simulink model "eom"  (R2021b)
settings: Solver=ode4  StartTime=0.0  StopTime=100  RelTol=1e-3  EnableMultiTasking=on
PreLoadFcn:
  | PARAMETROS
values from neighbouring files (symbols this model uses):
  b = 0.353    [PARAMETROS.m]    (also in forandtor.m; forandtorPARAM.m)
  CDfront = 0.5    [PARAMETROS.m]    (also in forandtor.m; forandtorPARAM.m)
  CDlat = 0.75    [PARAMETROS.m]    (also in forandtor.m; forandtorPARAM.m)
  CLa = 1    [PARAMETROS.m]    (also in forandtor.m; forandtorPARAM.m)
  CLp = 5    [PARAMETROS.m]    (also in forandtor.m; forandtorPARAM.m)
  CMdeltae = 1    [PARAMETROS.m]    (also in forandtor.m; forandtorPARAM.m)
  CMfq = 1    [PARAMETROS.m]    (also in forandtor.m; forandtorPARAM.m)
  CMw = 10    [PARAMETROS.m]    (also in forandtor.m; forandtorPARAM.m)
  CNdeltar = 1    [PARAMETROS.m]    (also in forandtor.m; forandtorPARAM.m)
  CNfr = 1    [PARAMETROS.m]    (also in forandtor.m; forandtorPARAM.m)
  CNv = 10    [PARAMETROS.m]    (also in forandtor.m; forandtorPARAM.m)
  fullt = 600    [PARAMETROS.m]    (also in forandtor.m; forandtorPARAM.m)
  g = 9.81    [PARAMETROS.m]    (also in eom1.m; eom1PARAM.m)
  Ix = 0.468    [PARAMETROS.m]    (also in eom1.m; eom1PARAM.m)
  Iy = 90.8    [PARAMETROS.m]    (also in eom1.m; eom1PARAM.m)
  Iz = Iy    (= 90.8)    [PARAMETROS.m]    (also in eom1.m; eom1PARAM.m)
  m = 85.3    [PARAMETROS.m]    (also in eom1.m; eom1PARAM.m)
  Sfront = 0.0127    [PARAMETROS.m]    (also in forandtor.m; forandtorPARAM.m)
  Slat = 1.2049    [PARAMETROS.m]    (also in forandtor.m; forandtorPARAM.m)
  Sstab = 0.45    [PARAMETROS.m]    (also in forandtor.m; forandtorPARAM.m)
  Swing = 0.4525    [PARAMETROS.m]    (also in forandtor.m; forandtorPARAM.m)
libraries: aerolibanim x6, aerolibatmos2 x3
(part 1 of 2)
settings Model: Creator=verti  LastModifiedBy=patri
settings SolverCC: MaxConsecutiveMinStep=0.1  ZeroCrossAlgorithm=Adaptive  AlgebraicLoopSolver=TrustRegion  AutoInsertRateTranBlk=on
settings DataIOCC: LimitDataPoints=on  ReturnWorkspaceOutputs=off
settings OptimizationCC: LifeSpan=inf
settings DebuggingCC: MultiTaskRateTransMsg=warning  AllowSymbolicDim=off  SFUnexpectedBacktrackingDiag=warning  SFNoUnconditionalDefaultTransitionDiag=warning  SFExecutionAtInitializationDiag=none  SFMachineParentedDataDiag=warning  ArithmeticOperatorsInVariantConditions=warning
settings ModelReferenceCC: PropagateSignalLabelsOutOfModel=off
settings SFSimCC: SimUseLocalCustomCode=off  CustomCodeUndefinedFunction=UseInterfaceOnly
settings RTWCC: RTWUseLocalCustomCode=off
settings CodeAppCC: StateflowObjectComments=on
settings GRTTargetCC: TargetLangStandard=C89/C90 (ANSI)
settings ConfigComp: CovMetricSettings=dw  CovSaveCumulativeToWorkspaceVar=on  CovSaveSingleToWorkspaceVar=on  CovExternalEMLEnable=off

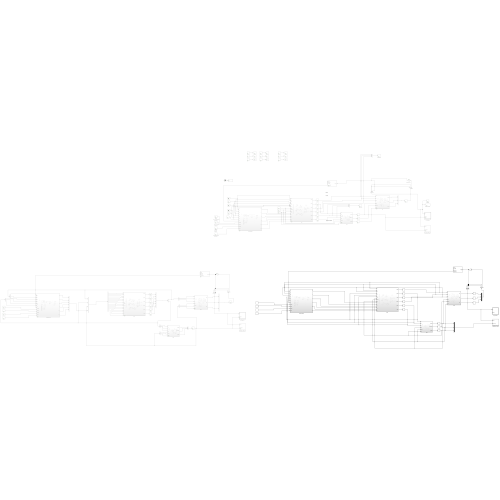
[thumbnail: Simulink's stored preview of the top-level diagram]
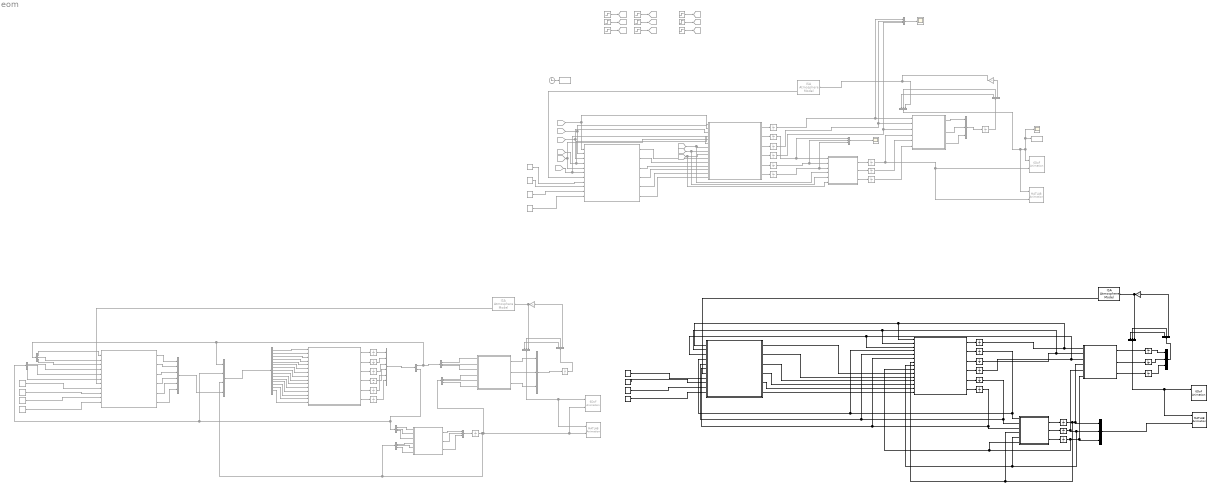
== system eom ==
  note: x,y,z
  note: Ángulos de Euler
  note: P,Q,R
  note: U,V,W
  Animación para ver la posición : aerolibanim/6DoF Animation  Commented=on  u1=[-1000 1000 -1000 1000 0 1300]  u2=0.1  u3=150.0  u4=[4000 0 -5000]  u5=Fixed position  u6=[2000 500 -3150]  u7=10  u8=on
  Animación para ver la posición1 : aerolibanim/6DoF Animation  Commented=on  u1=[-1000 1000 -1000 1000 0 1300]  u2=0.1  u3=150.0  u4=[4000 0 -5000]  u5=Fixed position  u6=[2000 500 -3150]  u7=10  u8=on
  Animación para ver la posición2 : aerolibanim/6DoF Animation  u1=[-1000 1000 -1000 1000 0 1300]  u2=0.1  u3=150.0  u4=[4000 0 -5000]  u5=Fixed position  u6=[2000 500 -3150]  u7=10  u8=on
  Animación para ver ángulos de euler : aerolibanim/MATLAB Animation  Tag=Matlab Animation 6 DOF  Commented=on  Vehicles=1  Geometries='astredwedge.mat'  BoundingBoxCoordinates=[-50,50,-50,50,-50,50]  CameraOffset=[-150,-50,0]  CameraViewAngle=3  SampleTime=0.2  FigurePosition=[1.386000e+02,5.322000e+02,368,2.696000e+02]
      settings: SourceProductBaseCode=AE
  Animación para ver ángulos de euler1 : aerolibanim/MATLAB Animation  Tag=Matlab Animation 6 DOF  Commented=on  Vehicles=1  Geometries='astredwedge.mat'  BoundingBoxCoordinates=[-50,50,-50,50,-50,50]  CameraOffset=[-150,-50,0]  CameraViewAngle=3  SampleTime=0.2  FigurePosition=[1.386000e+02,5.322000e+02,368,2.696000e+02]
      settings: SourceProductBaseCode=AE
  Animación para ver ángulos de euler2 : aerolibanim/MATLAB Animation  Tag=Matlab Animation 6 DOF  Vehicles=1  Geometries='astredwedge.mat'  BoundingBoxCoordinates=[-50,50,-50,50,-50,50]  CameraOffset=[-150,-50,0]  CameraViewAngle=3  SampleTime=0.2  FigurePosition=[1.386000e+02,5.322000e+02,368,2.696000e+02]
      settings: SourceProductBaseCode=AE
  Clock : Clock  Commented=on
  Constant1 : Constant  Value=0.1
  Constant2 : Constant  Commented=on  Value=0.1
  Constant3 : Constant  Commented=on  Value=0
  Constant4 : Constant  Commented=on  Value=0
  Constant5 : Constant  Commented=on
  Constant6 : Constant  Value=0
  Constant7 : Constant  Value=0
  Constant8 : Constant
  Demux{,1..2,5..9} (8 alike) : Demux  Commented=on  Outputs=3
  Demux18 : Demux  Outputs=3
  Demux3 : Demux  Commented=on  Outputs=15
  Demux4 : Demux  Commented=on  Outputs=2
  From1 : From  Commented=on  GotoTag=phi
  From2 : From  Commented=on  GotoTag=psi
  From3 : From  Commented=on  GotoTag=P
  From4 : From  Commented=on  GotoTag=Q
  From5 : From  Commented=on  GotoTag=R
  From6 : From  Commented=on  GotoTag=U
  From7 : From  Commented=on  GotoTag=W
  From8 : From  Commented=on  GotoTag=V
  From9 : From  Commented=on  GotoTag=theta
  Gain : Gain  Commented=on  Gain=-1
  Gain1 : Gain  Gain=-1
  Goto : Goto  Commented=on  GotoTag=U
  Goto1 : Goto  Commented=on  GotoTag=V
  Goto2 : Goto  Commented=on  GotoTag=W
  Goto3 : Goto  Commented=on  GotoTag=P
  Goto4 : Goto  Commented=on  GotoTag=Q
  Goto5 : Goto  Commented=on  GotoTag=R
  Goto6 : Goto  Commented=on  GotoTag=phi
  Goto7 : Goto  Commented=on  GotoTag=theta
  Goto8 : Goto  Commented=on  GotoTag=psi
  ISA Atmosphere Model : aerolibatmos2/ISA Atmosphere Model  Commented=on  custom=off  g=9.80665  gamma=1.4  R=287.0531  L=0.0065  h_trop=11000  h_strat=20000  rho0=1.225  P0=101325  T0=288.15  h0=0
  ISA Atmosphere Model1 : aerolibatmos2/ISA Atmosphere Model  custom=off  g=9.80665  gamma=1.4  R=287.0531  L=0.0065  h_trop=11000  h_strat=20000  rho0=1.225  P0=101325  T0=288.15  h0=0
  ISA Atmosphere Model2 : aerolibatmos2/ISA Atmosphere Model  Commented=on  custom=off  g=9.80665  gamma=1.4  R=287.0531  L=0.0065  h_trop=11000  h_strat=20000  rho0=1.225  P0=101325  T0=288.15  h0=0
  Integrator{,3..7,11,13..17} (12 alike) : Integrator  Commented=on  InitialCondition=[200,0,0,0,0,0]
  Integrator{1,8..9,12} (4 alike) : Integrator  Commented=on  InitialCondition=[0,0,0]
  Integrator10 : Integrator  Commented=on  InitialCondition=[0,0,-3000]
  Integrator18 : Integrator  InitialCondition=[0,0,-3000]
  Integrator{19,21..25} (6 alike) : Integrator  InitialCondition=[200,0,0,0,0,0]
  Integrator2 : Integrator  Commented=on  InitialCondition=[0,0,-3000]
  Integrator20 : Integrator  InitialCondition=[0,0,0]
  Integrator26 : Integrator  InitialCondition=[0,0,0]
  Integrator27 : Integrator  InitialCondition=[0,0,0]
  Integrator28 : Integrator  InitialCondition=[0,0,-3000]
  Integrator29 : Integrator  InitialCondition=[0,0,-3000]
  Inversión eje z : Gain  Commented=on  Gain=-1
  Momentos : Scope  Commented=on
  Mux{,2..3,5,7..9} (7 alike) : Mux  Commented=on  Inputs=3
  Mux1 : Mux  Commented=on  Inputs=6
  Mux10 : Mux  Inputs=3
  Mux11 : Mux  Inputs=3
  Mux14 : Mux  Inputs=3
  Mux4 : Mux  Commented=on
  Mux6 : Mux  Commented=on  Inputs=6
  Palanca de gases Empuje1 : Constant  Commented=on
  Step{,1..8} (9 alike) : Step  Commented=on  SampleTime=0
  To Workspace : ToWorkspace  Commented=on  VariableName=t  SampleTime=-1
  Vector posición : ToWorkspace  Commented=on  VariableName=posicion  SampleTime=-1
      settings: Decimation=2
  Velocidad : Scope  Commented=on
  delta timon profundidad cabeceo1 : Constant  Commented=on  Value=0.1
  deltaa alerones balance1 : Constant  Commented=on  Value=0
  deltar Timon vertical guiñada1 : Constant  Commented=on  Value=0
  eom : Subsystem  Commented=on
  eom1 : Subsystem  Commented=on  ClipboardFcn=PARAMETROS
  eom2 : Subsystem  ClipboardFcn=PARAMETROS
  forcesandtorq : Subsystem  Commented=on
  forcesandtorq1 : Subsystem  Commented=on  ClipboardFcn=PARAMETROS
  forcesandtorq2 : Subsystem  ClipboardFcn=PARAMETROS
  posición : Scope  Commented=on
  rang : Subsystem  Commented=on
  rang1 : Subsystem  Commented=on
  rang2 : Subsystem
  rtra : Subsystem  Commented=on
  rtra1 : Subsystem  Commented=on
  rtra2 : Subsystem
  wires:
  Clock/1 -> To Workspace/1
  Integrator1/1 -> rtra/4(phi), Animación para ver ángulos de euler/2, Animación para ver la posición/2
  Integrator2/1 -> Demux1/1
  Demux1/3 -> Inversión eje z/1
  Inversión eje z/1 -> Mux2/3, ISA Atmosphere Model/1
  ISA Atmosphere Model/4 -> forcesandtorq/7(ro)
  Demux1/1 -> Mux2/1
  Demux1/2 -> Mux2/2
  Mux2/1 -> posición/1, Vector posición/1, Animación para ver la posición/1, Animación para ver ángulos de euler/1
  delta timon profundidad cabeceo1/1 -> forcesandtorq/8(deltae)
  deltar Timon vertical guiñada1/1 -> forcesandtorq/9(deltar)
  deltaa alerones balance1/1 -> forcesandtorq/10(deltaa)
  Palanca de gases Empuje1/1 -> forcesandtorq/11(pgas)
  forcesandtorq/6(N) -> eom/15(N)
  forcesandtorq/5(M) -> eom/14(M)
  forcesandtorq/4(L) -> eom/13(L)
  forcesandtorq/3(Z) -> eom/12(Z)
  forcesandtorq/2(Y) -> eom/11(Y)
  forcesandtorq/1(X) -> eom/10(X)
  rtra/1(xdot) -> Mux5/1
  rtra/2(ydot) -> Mux5/2
  rtra/3(zdot) -> Mux5/3
  Mux5/1 -> Integrator2/1
  Step5/1 -> Goto5/1
  Step2/1 -> Goto2/1
  Step1/1 -> Goto1/1
  Step4/1 -> Goto4/1
  Step3/1 -> Goto3/1
  Step/1 -> Goto/1
  From6/1 -> forcesandtorq/1(U), eom/1(U)
  From8/1 -> forcesandtorq/2(V), eom/2(V)
  From7/1 -> forcesandtorq/3(W), eom/3(W)
  eom/1(udot) -> Integrator/1
  eom/2(pdot) -> Integrator3/1
  eom/3(vdot) -> Integrator4/1
  eom/6(rdot) -> Integrator7/1
  eom/5(qdot) -> Integrator6/1
  eom/4(wdot) -> Integrator5/1
  Integrator5/1 -> Mux/3, rtra/3(W)
  Integrator4/1 -> Mux/2, rtra/2(V)
  Integrator/1 -> Mux/1, rtra/1(U)
  Mux/1 -> Velocidad/1
  From3/1 -> eom/4(P), forcesandtorq/4(P)
  From4/1 -> forcesandtorq/5(Q), eom/5(Q)
  From5/1 -> eom/6(R), forcesandtorq/6(R)
  Integrator7/1 -> Mux3/3, rang/3(R)
  Integrator6/1 -> Mux3/2, rang/2(Q)
  Integrator3/1 -> Mux3/1, rang/1(P)
  Mux3/1 -> Momentos/1
  Step7/1 -> Goto7/1
  Step8/1 -> Goto8/1
  Step6/1 -> Goto6/1
  From1/1 -> rang/4(phi), eom/7(phi)
  From9/1 -> rang/5(theta), eom/8(theta)
  From2/1 -> rang/6(psi), eom/9(psi)
  rang/1(phidot) -> Integrator1/1
  rang/2(thetadot) -> Integrator8/1
  rang/3(psidot) -> Integrator9/1
  Integrator8/1 -> rtra/5(theta)
  Integrator9/1 -> rtra/6(psi)
  Demux/1 -> forcesandtorq1/1(U)
  Demux/2 -> forcesandtorq1/2(V)
  Demux/3 -> forcesandtorq1/3(W)
  Demux2/1 -> forcesandtorq1/4(P)
  Demux2/2 -> forcesandtorq1/5(Q)
  Demux2/3 -> forcesandtorq1/6(R)
  Constant2/1 -> forcesandtorq1/8(deltae)
  Constant3/1 -> forcesandtorq1/9(deltar)
  Constant4/1 -> forcesandtorq1/10(deltaa)
  Constant5/1 -> forcesandtorq1/11(pgas)
  forcesandtorq1/1(X) -> Mux1/1
  forcesandtorq1/2(Y) -> Mux1/2
  forcesandtorq1/3(Z) -> Mux1/3
  forcesandtorq1/4(L) -> Mux1/4
  forcesandtorq1/5(M) -> Mux1/5
  forcesandtorq1/6(N) -> Mux1/6
  Mux1/1 -> Mux4/4
  Demux3/1 -> eom1/1(U)
  Demux3/2 -> eom1/2(V)
  Demux3/3 -> eom1/3(W)
  Demux3/4 -> eom1/4(P)
  Demux3/5 -> eom1/5(Q)
  Demux3/6 -> eom1/6(R)
  Demux3/7 -> eom1/7(phi)
  Demux3/8 -> eom1/8(theta)
  Demux3/9 -> eom1/9(psi)
  Demux3/10 -> eom1/10(X)
  Demux3/11 -> eom1/11(Y)
  Demux3/12 -> eom1/12(Z)
  Demux3/13 -> eom1/13(L)
  Demux3/14 -> eom1/14(M)
  Demux3/15 -> eom1/15(N)
  Mux4/1 -> Demux3/1
  Demux5/1 -> rtra1/1(U)
  Demux5/2 -> rtra1/2(V)
  Demux5/3 -> rtra1/3(W)
  Demux6/1 -> rtra1/4(phi)
  Demux6/2 -> rtra1/5(theta)
  Demux6/3 -> rtra1/6(psi)
  Demux7/1 -> rang1/1(P)
  Demux7/2 -> rang1/2(Q)
  Demux7/3 -> rang1/3(R)
  Demux8/1 -> rang1/4(phi)
  Demux8/2 -> rang1/5(theta)
  Demux8/3 -> rang1/6(psi)
  rang1/1(phidot) -> Mux7/1
  rang1/2(thetadot) -> Mux7/2
  rang1/3(psidot) -> Mux7/3
  Mux7/1 -> Integrator12/1
  rtra1/1(xdot) -> Mux9/1
  rtra1/2(ydot) -> Mux9/2
  rtra1/3(zdot) -> Mux9/3
  Integrator10/1 -> Demux9/1
  Demux9/3 -> Gain/1
  Gain/1 -> ISA Atmosphere Model2/1, Mux8/3
  ISA Atmosphere Model2/4 -> forcesandtorq1/7(ro)
  Demux9/2 -> Mux8/2
  Demux9/1 -> Mux8/1
  Mux8/1 -> Animación para ver ángulos de euler1/1, Animación para ver la posición1/1
  Integrator12/1 -> Demux8/1, Mux4/3, Animación para ver ángulos de euler1/2, Animación para ver la posición1/2, Demux6/1
  Demux4/1 -> Mux4/1, Demux/1, Demux5/1
  Demux4/2 -> Mux4/2, Demux2/1, Demux7/1
  Mux9/1 -> Integrator10/1
  eom1/4(wdot) -> Integrator14/1
  eom1/3(vdot) -> Integrator15/1
  eom1/2(pdot) -> Integrator11/1
  eom1/1(udot) -> Integrator13/1
  eom1/5(qdot) -> Integrator16/1
  eom1/6(rdot) -> Integrator17/1
  Integrator13/1 -> Mux6/1
  Integrator11/1 -> Mux6/2
  Integrator15/1 -> Mux6/3
  Integrator14/1 -> Mux6/4
  Integrator16/1 -> Mux6/5
  Integrator17/1 -> Mux6/6
  Mux6/1 -> Demux4/1
  eom2/4(wdot) -> Integrator22/1
  eom2/1(udot) -> Integrator21/1
  eom2/6(rdot) -> Integrator25/1
  Constant8/1 -> forcesandtorq2/11(pgas)
  Constant7/1 -> forcesandtorq2/10(deltaa)
  eom2/2(pdot) -> Integrator19/1
  Integrator24/1 -> eom2/5(Q), forcesandtorq2/5(Q), rang2/2(Q)
  Constant1/1 -> forcesandtorq2/8(deltae)
  Gain1/1 -> ISA Atmosphere Model1/1, Mux14/3
  Demux18/1 -> Mux14/1
  Mux14/1 -> Animación para ver ángulos de euler2/1, Animación para ver la posición2/1
  ISA Atmosphere Model1/4 -> forcesandtorq2/7(ro)
  Integrator19/1 -> eom2/4(P), forcesandtorq2/4(P), rang2/1(P)
  Integrator25/1 -> eom2/6(R), forcesandtorq2/6(R), rang2/3(R)
  eom2/3(vdot) -> Integrator23/1
  eom2/5(qdot) -> Integrator24/1
  Constant6/1 -> forcesandtorq2/9(deltar)
  Demux18/2 -> Mux14/2
  Demux18/3 -> Gain1/1
  forcesandtorq2/1(X) -> eom2/10(X)
  forcesandtorq2/2(Y) -> eom2/11(Y)
  forcesandtorq2/3(Z) -> eom2/12(Z)
  forcesandtorq2/4(L) -> eom2/13(L)
  forcesandtorq2/5(M) -> eom2/14(M)
  forcesandtorq2/6(N) -> eom2/15(N)
  rang2/2(thetadot) -> Integrator26/1
  rang2/3(psidot) -> Integrator27/1
  rang2/1(phidot) -> Integrator20/1
  Integrator20/1 -> rang2/4(phi), eom2/7(phi), rtra2/4(phi), Mux10/1
  Integrator26/1 -> rtra2/5(theta), rang2/5(theta), eom2/8(theta), Mux10/2
  Integrator27/1 -> rang2/6(psi), eom2/9(psi), rtra2/6(psi), Mux10/3
  Mux10/1 -> Animación para ver ángulos de euler2/2
  Integrator21/1 -> eom2/1(U), forcesandtorq2/1(U), rtra2/1(U)
  Integrator23/1 -> eom2/2(V), forcesandtorq2/2(V), rtra2/2(V)
  Integrator22/1 -> eom2/3(W), forcesandtorq2/3(W), rtra2/3(W)
  rtra2/3(zdot) -> Integrator29/1
  rtra2/2(ydot) -> Integrator28/1
  rtra2/1(xdot) -> Integrator18/1
  Integrator18/1 -> Mux11/1
  Integrator28/1 -> Mux11/2
  Integrator29/1 -> Mux11/3
  Mux11/1 -> Demux18/1

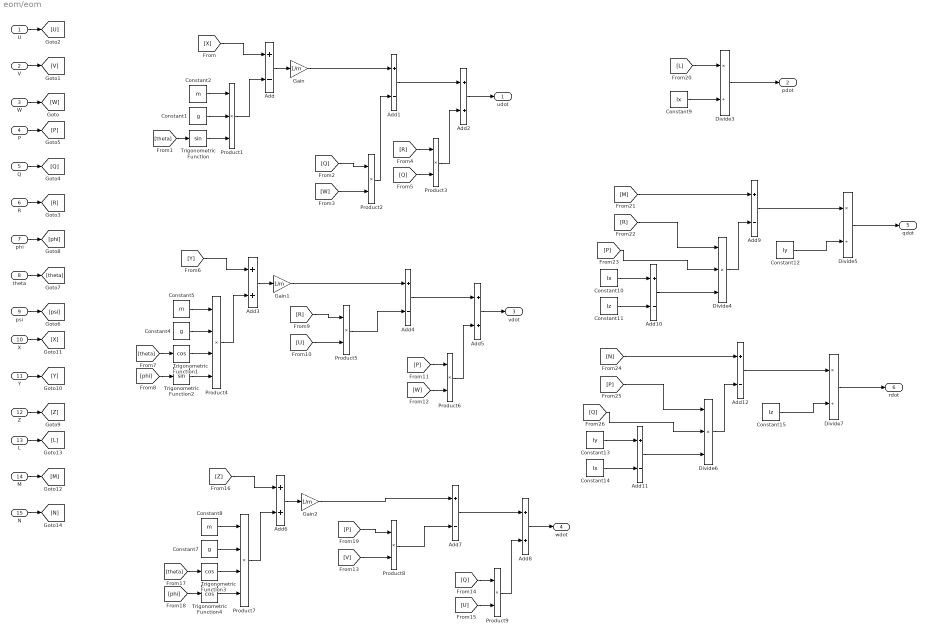
== system eom/eom ==
  U : Inport
  V : Inport  Port=2
  W : Inport  Port=3
  P : Inport  Port=4
  Q : Inport  Port=5
  R : Inport  Port=6
  phi : Inport  Port=7
  theta : Inport  Port=8
  psi : Inport  Port=9
  X : Inport  Port=10
  Y : Inport  Port=11
  Z : Inport  Port=12
  L : Inport  Port=13
  M : Inport  Port=14
  N : Inport  Port=15
  Add{,1,4,7,9..12} (8 alike) : Sum  Inputs=+-
  Add{2..3,5..6,8} (5 alike) : Sum
  Constant1 : Constant  Value=g
  Constant10 : Constant  Value=Ix
  Constant11 : Constant  Value=Iz
  Constant12 : Constant  Value=Iy
  Constant13 : Constant  Value=Iy
  Constant14 : Constant  Value=Ix
  Constant15 : Constant  Value=Iz
  Constant2 : Constant  Value=m
  Constant4 : Constant  Value=g
  Constant5 : Constant  Value=m
  Constant7 : Constant  Value=g
  Constant8 : Constant  Value=m
  Constant9 : Constant  Value=Ix
  Divide3 : Product  Inputs=*/
  Divide4 : Product  Inputs=3
  Divide5 : Product  Inputs=*/
  Divide6 : Product  Inputs=3
  Divide7 : Product  Inputs=*/
  Gain : Gain  Gain=1/m
  Gain1 : Gain  Gain=1/m
  Gain2 : Gain  Gain=1/m
  Product1 : Product  Inputs=3
  Product{2..3,5..6,8..9} (6 alike) : Product
  Product4 : Product  Inputs=4
  Product7 : Product  Inputs=4
  Trigonometric Function : Trigonometry
  Trigonometric Function1 : Trigonometry  Operator=cos
  Trigonometric Function2 : Trigonometry
  Trigonometric Function3 : Trigonometry  Operator=cos
  Trigonometric Function4 : Trigonometry  Operator=cos
  udot : Outport
  pdot : Outport  Port=2
  vdot : Outport  Port=3
  wdot : Outport  Port=4
  qdot : Outport  Port=5
  rdot : Outport  Port=6
  wires:
  W/1 -> [W]
  V/1 -> [V]
  U/1 -> [U]
  Q/1 -> [Q]
  P/1 -> [P]
  R/1 -> [R]
  theta/1 -> [theta]
  phi/1 -> [phi]
  psi/1 -> [psi]
  Z/1 -> [Z]
  X/1 -> [X]
  Y/1 -> [Y]
  N/1 -> [N]
  M/1 -> [M]
  L/1 -> [L]
  [X] -> Add/1
  [theta] -> Trigonometric Function/1
  Trigonometric Function/1 -> Product1/3
  Constant2/1 -> Product1/1
  Constant1/1 -> Product1/2
  Product1/1 -> Add/2
  Add/1 -> Gain/1
  Gain/1 -> Add1/1
  [W] -> Product2/2
  [Q] -> Product2/1
  Product2/1 -> Add1/2
  Add1/1 -> Add2/1
  Add2/1 -> udot/1
  [Q] -> Product3/2
  [R] -> Product3/1
  Product3/1 -> Add2/2
  [Y] -> Add3/1
  Trigonometric Function1/1 -> Product4/3
  Product4/1 -> Add3/2
  Add3/1 -> Gain1/1
  Constant5/1 -> Product4/1
  [theta] -> Trigonometric Function1/1
  Constant4/1 -> Product4/2
  [phi] -> Trigonometric Function2/1
  Trigonometric Function2/1 -> Product4/4
  Gain1/1 -> Add4/1
  [U] -> Product5/2
  [R] -> Product5/1
  Product5/1 -> Add4/2
  Add4/1 -> Add5/1
  Add5/1 -> vdot/1
  [W] -> Product6/2
  Product6/1 -> Add5/2
  [P] -> Product6/1
  Trigonometric Function4/1 -> Product7/4
  Add8/1 -> wdot/1
  [P] -> Product8/1
  [V] -> Product8/2
  [Z] -> Add6/1
  [phi] -> Trigonometric Function4/1
  Add7/1 -> Add8/1
  Constant7/1 -> Product7/2
  [theta] -> Trigonometric Function3/1
  Trigonometric Function3/1 -> Product7/3
  [U] -> Product9/2
  Product7/1 -> Add6/2
  [Q] -> Product9/1
  Constant8/1 -> Product7/1
  Product8/1 -> Add7/2
  Add6/1 -> Gain2/1
  Gain2/1 -> Add7/1
  Product9/1 -> Add8/2
  [L] -> Divide3/1
  Constant9/1 -> Divide3/2
  Divide3/1 -> pdot/1
  [M] -> Add9/1
  Constant10/1 -> Add10/1
  Constant11/1 -> Add10/2
  Divide4/1 -> Add9/2
  Add10/1 -> Divide4/3
  [P] -> Divide4/2
  [R] -> Divide4/1
  Add9/1 -> Divide5/1
  Constant12/1 -> Divide5/2
  Divide5/1 -> qdot/1
  Divide7/1 -> rdot/1
  [N] -> Add12/1
  Add12/1 -> Divide7/1
  Constant14/1 -> Add11/2
  [P] -> Divide6/1
  Constant13/1 -> Add11/1
  Divide6/1 -> Add12/2
  Add11/1 -> Divide6/3
  [Q] -> Divide6/2
  Constant15/1 -> Divide7/2

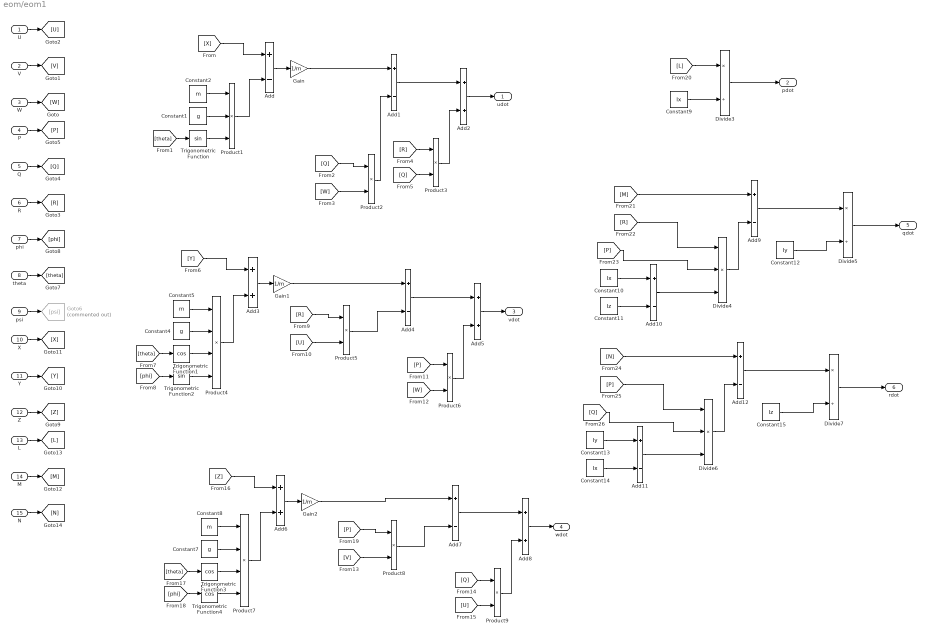
== system eom/eom1 ==
  U : Inport
  V : Inport  Port=2
  W : Inport  Port=3
  P : Inport  Port=4
  Q : Inport  Port=5
  R : Inport  Port=6
  phi : Inport  Port=7
  theta : Inport  Port=8
  psi : Inport  Port=9
  X : Inport  Port=10
  Y : Inport  Port=11
  Z : Inport  Port=12
  L : Inport  Port=13
  M : Inport  Port=14
  N : Inport  Port=15
  Add{,1,4,7,9..12} (8 alike) : Sum  Inputs=+-
  Add{2..3,5..6,8} (5 alike) : Sum
  Constant1 : Constant  Value=g
  Constant10 : Constant  Value=Ix
  Constant11 : Constant  Value=Iz
  Constant12 : Constant  Value=Iy
  Constant13 : Constant  Value=Iy
  Constant14 : Constant  Value=Ix
  Constant15 : Constant  Value=Iz
  Constant2 : Constant  Value=m
  Constant4 : Constant  Value=g
  Constant5 : Constant  Value=m
  Constant7 : Constant  Value=g
  Constant8 : Constant  Value=m
  Constant9 : Constant  Value=Ix
  Divide3 : Product  Inputs=*/
  Divide4 : Product  Inputs=3
  Divide5 : Product  Inputs=*/
  Divide6 : Product  Inputs=3
  Divide7 : Product  Inputs=*/
  Gain : Gain  Gain=1/m
  Gain1 : Gain  Gain=1/m
  Gain2 : Gain  Gain=1/m
  Goto6 : Goto  Commented=on  GotoTag=psi
  Product1 : Product  Inputs=3
  Product{2..3,5..6,8..9} (6 alike) : Product
  Product4 : Product  Inputs=4
  Product7 : Product  Inputs=4
  Trigonometric Function : Trigonometry
  Trigonometric Function1 : Trigonometry  Operator=cos
  Trigonometric Function2 : Trigonometry
  Trigonometric Function3 : Trigonometry  Operator=cos
  Trigonometric Function4 : Trigonometry  Operator=cos
  udot : Outport
  pdot : Outport  Port=2
  vdot : Outport  Port=3
  wdot : Outport  Port=4
  qdot : Outport  Port=5
  rdot : Outport  Port=6
  wires:
  W/1 -> [W]
  V/1 -> [V]
  U/1 -> [U]
  Q/1 -> [Q]
  P/1 -> [P]
  R/1 -> [R]
  theta/1 -> [theta]
  phi/1 -> [phi]
  psi/1 -> Goto6/1
  Z/1 -> [Z]
  X/1 -> [X]
  Y/1 -> [Y]
  N/1 -> [N]
  M/1 -> [M]
  L/1 -> [L]
  [X] -> Add/1
  [theta] -> Trigonometric Function/1
  Trigonometric Function/1 -> Product1/3
  Constant2/1 -> Product1/1
  Constant1/1 -> Product1/2
  Product1/1 -> Add/2
  Add/1 -> Gain/1
  Gain/1 -> Add1/1
  [W] -> Product2/2
  [Q] -> Product2/1
  Product2/1 -> Add1/2
  Add1/1 -> Add2/1
  Add2/1 -> udot/1
  [Q] -> Product3/2
  [R] -> Product3/1
  Product3/1 -> Add2/2
  [Y] -> Add3/1
  Trigonometric Function1/1 -> Product4/3
  Product4/1 -> Add3/2
  Add3/1 -> Gain1/1
  Constant5/1 -> Product4/1
  [theta] -> Trigonometric Function1/1
  Constant4/1 -> Product4/2
  [phi] -> Trigonometric Function2/1
  Trigonometric Function2/1 -> Product4/4
  Gain1/1 -> Add4/1
  [U] -> Product5/2
  [R] -> Product5/1
  Product5/1 -> Add4/2
  Add4/1 -> Add5/1
  Add5/1 -> vdot/1
  [W] -> Product6/2
  Product6/1 -> Add5/2
  [P] -> Product6/1
  Trigonometric Function4/1 -> Product7/4
  Add8/1 -> wdot/1
  [P] -> Product8/1
  [V] -> Product8/2
  [Z] -> Add6/1
  [phi] -> Trigonometric Function4/1
  Add7/1 -> Add8/1
  Constant7/1 -> Product7/2
  [theta] -> Trigonometric Function3/1
  Trigonometric Function3/1 -> Product7/3
  [U] -> Product9/2
  Product7/1 -> Add6/2
  [Q] -> Product9/1
  Constant8/1 -> Product7/1
  Product8/1 -> Add7/2
  Add6/1 -> Gain2/1
  Gain2/1 -> Add7/1
  Product9/1 -> Add8/2
  [L] -> Divide3/1
  Constant9/1 -> Divide3/2
  Divide3/1 -> pdot/1
  [M] -> Add9/1
  Constant10/1 -> Add10/1
  Constant11/1 -> Add10/2
  Divide4/1 -> Add9/2
  Add10/1 -> Divide4/3
  [P] -> Divide4/2
  [R] -> Divide4/1
  Add9/1 -> Divide5/1
  Constant12/1 -> Divide5/2
  Divide5/1 -> qdot/1
  Divide7/1 -> rdot/1
  [N] -> Add12/1
  Add12/1 -> Divide7/1
  Constant14/1 -> Add11/2
  [P] -> Divide6/1
  Constant13/1 -> Add11/1
  Divide6/1 -> Add12/2
  Add11/1 -> Divide6/3
  [Q] -> Divide6/2
  Constant15/1 -> Divide7/2

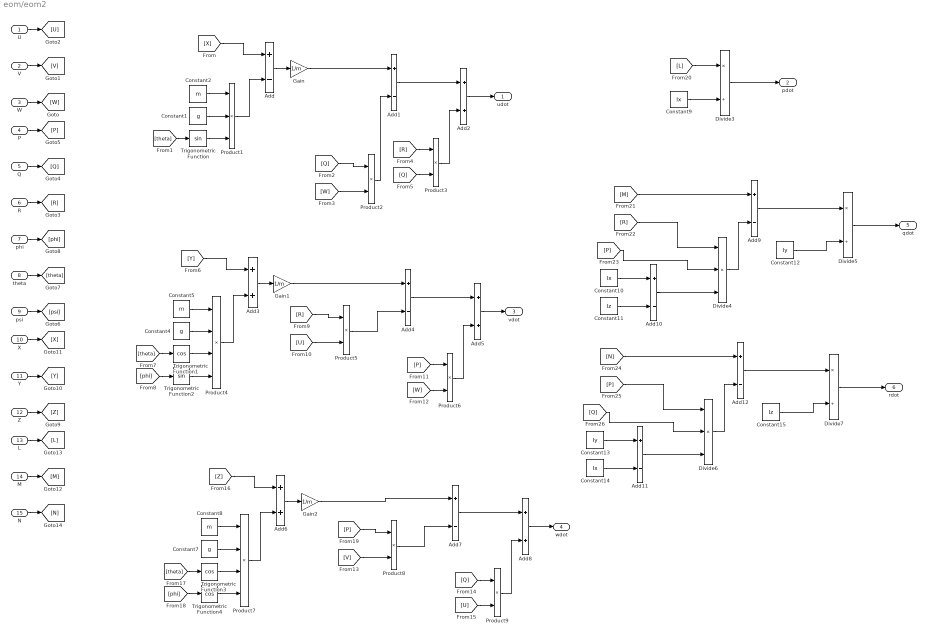
== system eom/eom2 ==
  U : Inport
  V : Inport  Port=2
  W : Inport  Port=3
  P : Inport  Port=4
  Q : Inport  Port=5
  R : Inport  Port=6
  phi : Inport  Port=7
  theta : Inport  Port=8
  psi : Inport  Port=9
  X : Inport  Port=10
  Y : Inport  Port=11
  Z : Inport  Port=12
  L : Inport  Port=13
  M : Inport  Port=14
  N : Inport  Port=15
  Add{,1,4,7,9..12} (8 alike) : Sum  Inputs=+-
  Add{2..3,5..6,8} (5 alike) : Sum
  Constant1 : Constant  Value=g
  Constant10 : Constant  Value=Ix
  Constant11 : Constant  Value=Iz
  Constant12 : Constant  Value=Iy
  Constant13 : Constant  Value=Iy
  Constant14 : Constant  Value=Ix
  Constant15 : Constant  Value=Iz
  Constant2 : Constant  Value=m
  Constant4 : Constant  Value=g
  Constant5 : Constant  Value=m
  Constant7 : Constant  Value=g
  Constant8 : Constant  Value=m
  Constant9 : Constant  Value=Ix
  Divide3 : Product  Inputs=*/
  Divide4 : Product  Inputs=3
  Divide5 : Product  Inputs=*/
  Divide6 : Product  Inputs=3
  Divide7 : Product  Inputs=*/
  Gain : Gain  Gain=1/m
  Gain1 : Gain  Gain=1/m
  Gain2 : Gain  Gain=1/m
  Product1 : Product  Inputs=3
  Product{2..3,5..6,8..9} (6 alike) : Product
  Product4 : Product  Inputs=4
  Product7 : Product  Inputs=4
  Trigonometric Function : Trigonometry
  Trigonometric Function1 : Trigonometry  Operator=cos
  Trigonometric Function2 : Trigonometry
  Trigonometric Function3 : Trigonometry  Operator=cos
  Trigonometric Function4 : Trigonometry  Operator=cos
  udot : Outport
  pdot : Outport  Port=2
  vdot : Outport  Port=3
  wdot : Outport  Port=4
  qdot : Outport  Port=5
  rdot : Outport  Port=6
  wires:
  W/1 -> [W]
  V/1 -> [V]
  U/1 -> [U]
  Q/1 -> [Q]
  P/1 -> [P]
  R/1 -> [R]
  theta/1 -> [theta]
  phi/1 -> [phi]
  psi/1 -> [psi]
  Z/1 -> [Z]
  X/1 -> [X]
  Y/1 -> [Y]
  N/1 -> [N]
  M/1 -> [M]
  L/1 -> [L]
  [X] -> Add/1
  [theta] -> Trigonometric Function/1
  Trigonometric Function/1 -> Product1/3
  Constant2/1 -> Product1/1
  Constant1/1 -> Product1/2
  Product1/1 -> Add/2
  Add/1 -> Gain/1
  Gain/1 -> Add1/1
  [W] -> Product2/2
  [Q] -> Product2/1
  Product2/1 -> Add1/2
  Add1/1 -> Add2/1
  Add2/1 -> udot/1
  [Q] -> Product3/2
  [R] -> Product3/1
  Product3/1 -> Add2/2
  [Y] -> Add3/1
  Trigonometric Function1/1 -> Product4/3
  Product4/1 -> Add3/2
  Add3/1 -> Gain1/1
  Constant5/1 -> Product4/1
  [theta] -> Trigonometric Function1/1
  Constant4/1 -> Product4/2
  [phi] -> Trigonometric Function2/1
  Trigonometric Function2/1 -> Product4/4
  Gain1/1 -> Add4/1
  [U] -> Product5/2
  [R] -> Product5/1
  Product5/1 -> Add4/2
  Add4/1 -> Add5/1
  Add5/1 -> vdot/1
  [W] -> Product6/2
  Product6/1 -> Add5/2
  [P] -> Product6/1
  Trigonometric Function4/1 -> Product7/4
  Add8/1 -> wdot/1
  [P] -> Product8/1
  [V] -> Product8/2
  [Z] -> Add6/1
  [phi] -> Trigonometric Function4/1
  Add7/1 -> Add8/1
  Constant7/1 -> Product7/2
  [theta] -> Trigonometric Function3/1
  Trigonometric Function3/1 -> Product7/3
  [U] -> Product9/2
  Product7/1 -> Add6/2
  [Q] -> Product9/1
  Constant8/1 -> Product7/1
  Product8/1 -> Add7/2
  Add6/1 -> Gain2/1
  Gain2/1 -> Add7/1
  Product9/1 -> Add8/2
  [L] -> Divide3/1
  Constant9/1 -> Divide3/2
  Divide3/1 -> pdot/1
  [M] -> Add9/1
  Constant10/1 -> Add10/1
  Constant11/1 -> Add10/2
  Divide4/1 -> Add9/2
  Add10/1 -> Divide4/3
  [P] -> Divide4/2
  [R] -> Divide4/1
  Add9/1 -> Divide5/1
  Constant12/1 -> Divide5/2
  Divide5/1 -> qdot/1
  Divide7/1 -> rdot/1
  [N] -> Add12/1
  Add12/1 -> Divide7/1
  Constant14/1 -> Add11/2
  [P] -> Divide6/1
  Constant13/1 -> Add11/1
  Divide6/1 -> Add12/2
  Add11/1 -> Divide6/3
  [Q] -> Divide6/2
  Constant15/1 -> Divide7/2

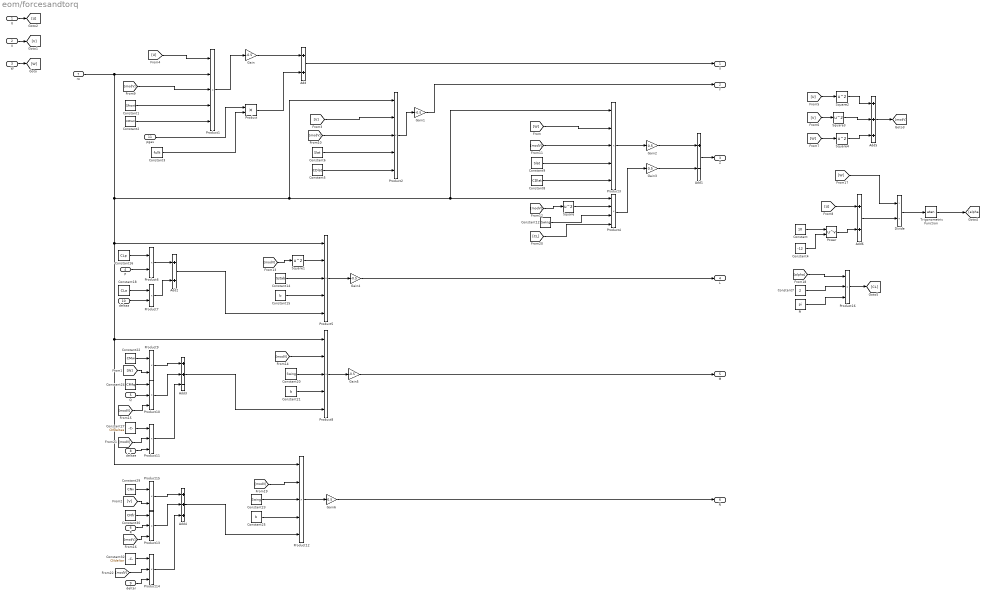
== system eom/forcesandtorq ==
  U : Inport
  V : Inport  Port=2
  W : Inport  Port=3
  P : Inport  Port=4
  Q : Inport  Port=5
  R : Inport  Port=6
  ro : Inport  Port=7
  deltae : Inport  Port=8
  deltar : Inport  Port=9
  deltaa : Inport  Port=10
  pgas : Inport  Port=11
  Add : Sum
  Add1 : Sum  Inputs=+-
  Add2 : Sum
  Add3 : Sum  Inputs=++-
  Add4 : Sum  Inputs=+++
  Add5 : Sum  Inputs=+++
  Add6 : Sum
  Constant : Constant  Value=10
  Constant1 : Constant  Value=Sfront
  Constant12 : Constant  Value=Swing
  Constant14 : Constant  Value=Sstab
  Constant15 : Constant  Value=b
  Constant16 : Constant  Value=CLp
  Constant18 : Constant  Value=CLa
  Constant2 : Constant  Value=CDfront
  Constant20 : Constant  Value=Swing
  Constant21 : Constant  Value=b
  Constant22 : Constant  Value=CMw
  Constant23 : Constant  Value=Swing
  Constant24 : Constant  Value=CMfq
  Constant25 : Constant  Value=b
  Constant27 : Constant  Value=CMdeltae
  Constant29 : Constant  Value=CNv
  Constant3 : Constant  Value=fullt
  Constant30 : Constant  Value=CNfr
  Constant32 : Constant  Value=CNdeltar
  Constant4 : Constant  Value=-12
  Constant5 : Constant  Value=CDlat
  Constant6 : Constant  Value=Slat
  Constant7 : Constant  Value=2
  Constant8 : Constant  Value=CDlat
  Constant9 : Constant  Value=Slat
  Divide : Product  Inputs=*/
  Gain{,1,4..6} (5 alike) : Gain  Gain=-0.5
  Gain2 : Gain  Gain=0.5
  Gain3 : Gain  Gain=0.5
  Pi : Constant  Value=pi  OutDataTypeStr=Inherit: Inherit via back propagation
  Power : Math  Operator=pow  SaturateOnIntegerOverflow=on
  Product{,6..7,9,15} (5 alike) : Product
  Product{1..3,5,8,12} (6 alike) : Product  Inputs=5
  Product{10..11,13..14,16} (5 alike) : Product  Inputs=3
  Product4 : Product  Inputs=4
  Square{,1..4} (5 alike) : Math  Operator=square  SaturateOnIntegerOverflow=on
  Trigonometric Function : Trigonometry  Operator=atan
  X : Outport
  Y : Outport  Port=2
  Z : Outport  Port=3
  L : Outport  Port=4
  M : Outport  Port=5
  N : Outport  Port=6
  wires:
  pgas/1 -> Product/1
  Product/1 -> Add/2
  Constant1/1 -> Product1/4
  Constant2/1 -> Product1/5
  Product1/1 -> Gain/1
  Gain/1 -> Add/1
  Constant3/1 -> Product/2
  Add/1 -> X/1
  Product2/1 -> Gain1/1
  Constant6/1 -> Product2/4
  [modV] -> Product2/3
  Constant5/1 -> Product2/5
  Gain1/1 -> Y/1
  [modV] -> Product3/3
  Constant9/1 -> Product3/4
  Constant8/1 -> Product3/5
  Product3/1 -> Gain2/1
  Gain2/1 -> Add1/1
  Product4/1 -> Gain3/1
  Gain3/1 -> Add1/2
  [modV] -> Square/1
  Square/1 -> Product4/2
  Constant12/1 -> Product4/3
  Add1/1 -> Z/1
  Square1/1 -> Product5/2
  [modV] -> Square1/1
  Constant14/1 -> Product5/3
  Constant15/1 -> Product5/4
  Constant16/1 -> Product6/1
  Constant18/1 -> Product7/1
  deltaa/1 -> Product7/2
  Product7/1 -> Add2/2
  Product6/1 -> Add2/1
  Add2/1 -> Product5/5
  Product5/1 -> Gain4/1
  Gain4/1 -> L/1
  Product8/1 -> Gain5/1
  [modV] -> Product8/2
  Constant20/1 -> Product8/3
  Constant21/1 -> Product8/4
  Constant22/1 -> Product9/1
  Constant24/1 -> Product10/1
  [modV] -> Product10/3
  Constant27/1 -> Product11/1
  Product9/1 -> Add3/1
  Product10/1 -> Add3/2
  Product11/1 -> Add3/3
  Add3/1 -> Product8/5
  Gain5/1 -> M/1
  deltae/1 -> Product11/3
  W/1 -> [W]
  [W] -> Product3/2
  [W] -> Product9/2
  P/1 -> Product6/2
  Q/1 -> Product10/2
  Product12/1 -> Gain6/1
  ro/1 -> Product12/1, Product8/1, Product5/1, Product4/1, Product3/1, Product2/1, Product1/2
  Constant23/1 -> Product12/3
  Constant25/1 -> Product12/4
  [V] -> Product15/2
  Constant30/1 -> Product13/1
  Product15/1 -> Add4/1
  Product14/1 -> Add4/3
  Constant32/1 -> Product14/1
  [modV] -> Product13/3
  [modV] -> Product14/2
  Constant29/1 -> Product15/1
  Product13/1 -> Add4/2
  Add4/1 -> Product12/5
  R/1 -> Product13/2
  deltar/1 -> Product14/3
  Gain6/1 -> N/1
  V/1 -> [V]
  [V] -> Product2/2
  U/1 -> [U]
  [U] -> Product1/1
  [W] -> Square4/1
  [V] -> Square3/1
  [U] -> Square2/1
  Square2/1 -> Add5/1
  Square3/1 -> Add5/2
  Square4/1 -> Add5/3
  Add5/1 -> [modV]
  [modV] -> Product1/3
  Constant4/1 -> Power/2
  Constant/1 -> Power/1
  Power/1 -> Add6/2
  [U] -> Add6/1
  Add6/1 -> Divide/2
  [W] -> Divide/1
  Divide/1 -> Trigonometric Function/1
  Trigonometric Function/1 -> [alpha]
  [alpha] -> Product16/1
  Constant7/1 -> Product16/2
  Pi/1 -> Product16/3
  Product16/1 -> [CL]
  [CL] -> Product4/4
  [modV] -> Product12/2
  [modV] -> Product11/2

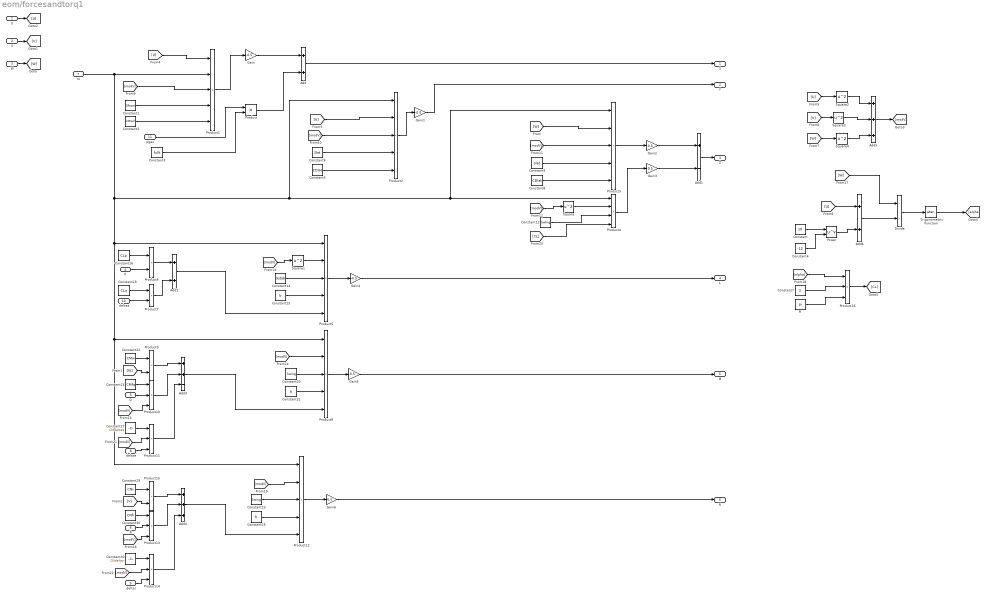
== system eom/forcesandtorq1 ==
  U : Inport
  V : Inport  Port=2
  W : Inport  Port=3
  P : Inport  Port=4
  Q : Inport  Port=5
  R : Inport  Port=6
  ro : Inport  Port=7
  deltae : Inport  Port=8
  deltar : Inport  Port=9
  deltaa : Inport  Port=10
  pgas : Inport  Port=11
  Add : Sum
  Add1 : Sum  Inputs=+-
  Add2 : Sum
  Add3 : Sum  Inputs=++-
  Add4 : Sum  Inputs=+++
  Add5 : Sum  Inputs=+++
  Add6 : Sum
  Constant : Constant  Value=10
  Constant1 : Constant  Value=Sfront
  Constant12 : Constant  Value=Swing
  Constant14 : Constant  Value=Sstab
  Constant15 : Constant  Value=b
  Constant16 : Constant  Value=CLp
  Constant18 : Constant  Value=CLa
  Constant2 : Constant  Value=CDfront
  Constant20 : Constant  Value=Swing
  Constant21 : Constant  Value=b
  Constant22 : Constant  Value=CMw
  Constant23 : Constant  Value=Swing
  Constant24 : Constant  Value=CMfq
  Constant25 : Constant  Value=b
  Constant27 : Constant  Value=CMdeltae
  Constant29 : Constant  Value=CNv
  Constant3 : Constant  Value=fullt
  Constant30 : Constant  Value=CNfr
  Constant32 : Constant  Value=CNdeltar
  Constant4 : Constant  Value=-12
  Constant5 : Constant  Value=CDlat
  Constant6 : Constant  Value=Slat
  Constant7 : Constant  Value=2
  Constant8 : Constant  Value=CDlat
  Constant9 : Constant  Value=Slat
  Divide : Product  Inputs=*/
  Gain{,1,4..6} (5 alike) : Gain  Gain=-0.5
  Gain2 : Gain  Gain=0.5
  Gain3 : Gain  Gain=0.5
  Pi : Constant  Value=pi  OutDataTypeStr=Inherit: Inherit via back propagation
  Power : Math  Operator=pow  SaturateOnIntegerOverflow=on
  Product{,6..7,9,15} (5 alike) : Product
  Product{1..3,5,8,12} (6 alike) : Product  Inputs=5
  Product{10..11,13..14,16} (5 alike) : Product  Inputs=3
  Product4 : Product  Inputs=4
  Square{,1..4} (5 alike) : Math  Operator=square  SaturateOnIntegerOverflow=on
  Trigonometric Function : Trigonometry  Operator=atan
  X : Outport
  Y : Outport  Port=2
  Z : Outport  Port=3
  L : Outport  Port=4
  M : Outport  Port=5
  N : Outport  Port=6
  wires:
  pgas/1 -> Product/1
  Product/1 -> Add/2
  Constant1/1 -> Product1/4
  Constant2/1 -> Product1/5
  Product1/1 -> Gain/1
  Gain/1 -> Add/1
  Constant3/1 -> Product/2
  Add/1 -> X/1
  Product2/1 -> Gain1/1
  Constant6/1 -> Product2/4
  [modV] -> Product2/3
  Constant5/1 -> Product2/5
  Gain1/1 -> Y/1
  [modV] -> Product3/3
  Constant9/1 -> Product3/4
  Constant8/1 -> Product3/5
  Product3/1 -> Gain2/1
  Gain2/1 -> Add1/1
  Product4/1 -> Gain3/1
  Gain3/1 -> Add1/2
  [modV] -> Square/1
  Square/1 -> Product4/2
  Constant12/1 -> Product4/3
  Add1/1 -> Z/1
  Square1/1 -> Product5/2
  [modV] -> Square1/1
  Constant14/1 -> Product5/3
  Constant15/1 -> Product5/4
  Constant16/1 -> Product6/1
  Constant18/1 -> Product7/1
  deltaa/1 -> Product7/2
  Product7/1 -> Add2/2
  Product6/1 -> Add2/1
  Add2/1 -> Product5/5
  Product5/1 -> Gain4/1
  Gain4/1 -> L/1
  Product8/1 -> Gain5/1
  [modV] -> Product8/2
  Constant20/1 -> Product8/3
  Constant21/1 -> Product8/4
  Constant22/1 -> Product9/1
  Constant24/1 -> Product10/1
  [modV] -> Product10/3
  Constant27/1 -> Product11/1
  Product9/1 -> Add3/1
  Product10/1 -> Add3/2
  Product11/1 -> Add3/3
  Add3/1 -> Product8/5
  Gain5/1 -> M/1
  deltae/1 -> Product11/3
  W/1 -> [W]
  [W] -> Product3/2
  [W] -> Product9/2
  P/1 -> Product6/2
  Q/1 -> Product10/2
  Product12/1 -> Gain6/1
  ro/1 -> Product12/1, Product8/1, Product5/1, Product4/1, Product3/1, Product2/1, Product1/2
  Constant23/1 -> Product12/3
  Constant25/1 -> Product12/4
  [V] -> Product15/2
  Constant30/1 -> Product13/1
  Product15/1 -> Add4/1
  Product14/1 -> Add4/3
  Constant32/1 -> Product14/1
  [modV] -> Product13/3
  [modV] -> Product14/2
  Constant29/1 -> Product15/1
  Product13/1 -> Add4/2
  Add4/1 -> Product12/5
  R/1 -> Product13/2
  deltar/1 -> Product14/3
  Gain6/1 -> N/1
  V/1 -> [V]
  [V] -> Product2/2
  U/1 -> [U]
  [U] -> Product1/1
  [W] -> Square4/1
  [V] -> Square3/1
  [U] -> Square2/1
  Square2/1 -> Add5/1
  Square3/1 -> Add5/2
  Square4/1 -> Add5/3
  Add5/1 -> [modV]
  [modV] -> Product1/3
  Constant4/1 -> Power/2
  Constant/1 -> Power/1
  Power/1 -> Add6/2
  [U] -> Add6/1
  Add6/1 -> Divide/2
  [W] -> Divide/1
  Divide/1 -> Trigonometric Function/1
  Trigonometric Function/1 -> [alpha]
  [alpha] -> Product16/1
  Constant7/1 -> Product16/2
  Pi/1 -> Product16/3
  Product16/1 -> [CL]
  [CL] -> Product4/4
  [modV] -> Product12/2
  [modV] -> Product11/2

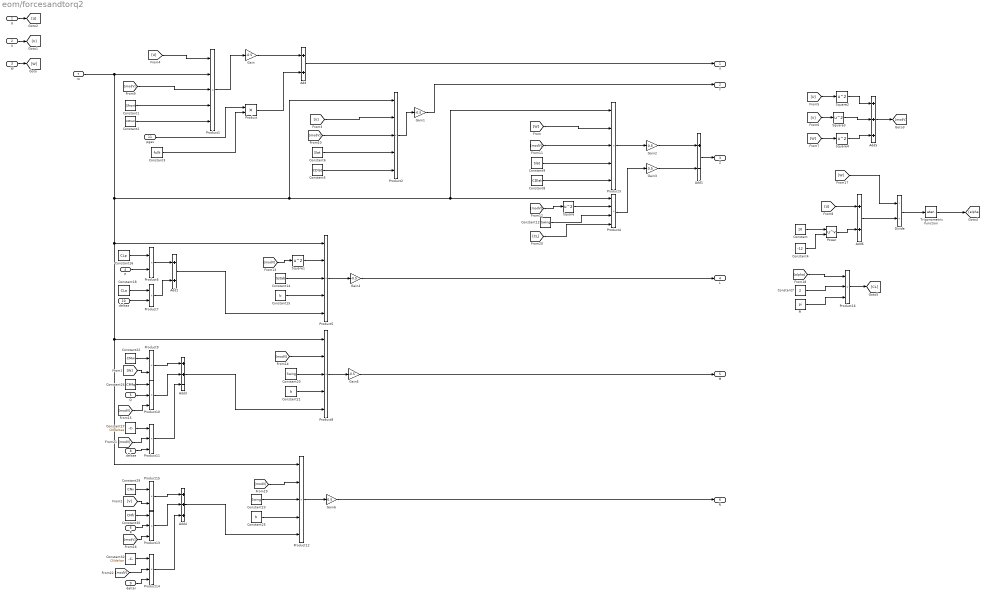
== system eom/forcesandtorq2 ==
  U : Inport
  V : Inport  Port=2
  W : Inport  Port=3
  P : Inport  Port=4
  Q : Inport  Port=5
  R : Inport  Port=6
  ro : Inport  Port=7
  deltae : Inport  Port=8
  deltar : Inport  Port=9
  deltaa : Inport  Port=10
  pgas : Inport  Port=11
  Add : Sum
  Add1 : Sum  Inputs=+-
  Add2 : Sum
  Add3 : Sum  Inputs=++-
  Add4 : Sum  Inputs=+++
  Add5 : Sum  Inputs=+++
  Add6 : Sum
  Constant : Constant  Value=10
  Constant1 : Constant  Value=Sfront
  Constant12 : Constant  Value=Swing
  Constant14 : Constant  Value=Sstab
  Constant15 : Constant  Value=b
  Constant16 : Constant  Value=CLp
  Constant18 : Constant  Value=CLa
  Constant2 : Constant  Value=CDfront
  Constant20 : Constant  Value=Swing
  Constant21 : Constant  Value=b
  Constant22 : Constant  Value=CMw
  Constant23 : Constant  Value=Swing
  Constant24 : Constant  Value=CMfq
  Constant25 : Constant  Value=b
  Constant27 : Constant  Value=CMdeltae
  Constant29 : Constant  Value=CNv
  Constant3 : Constant  Value=fullt
  Constant30 : Constant  Value=CNfr
  Constant32 : Constant  Value=CNdeltar
  Constant4 : Constant  Value=-12
  Constant5 : Constant  Value=CDlat
  Constant6 : Constant  Value=Slat
  Constant7 : Constant  Value=2
  Constant8 : Constant  Value=CDlat
  Constant9 : Constant  Value=Slat
  Divide : Product  Inputs=*/
  Gain{,1,4..6} (5 alike) : Gain  Gain=-0.5
  Gain2 : Gain  Gain=0.5
  Gain3 : Gain  Gain=0.5
  Pi : Constant  Value=pi  OutDataTypeStr=Inherit: Inherit via back propagation
  Power : Math  Operator=pow  SaturateOnIntegerOverflow=on
  Product{,6..7,9,15} (5 alike) : Product
  Product{1..3,5,8,12} (6 alike) : Product  Inputs=5
  Product{10..11,13..14,16} (5 alike) : Product  Inputs=3
  Product4 : Product  Inputs=4
  Square{,1..4} (5 alike) : Math  Operator=square  SaturateOnIntegerOverflow=on
  Trigonometric Function : Trigonometry  Operator=atan
  X : Outport
  Y : Outport  Port=2
  Z : Outport  Port=3
  L : Outport  Port=4
  M : Outport  Port=5
  N : Outport  Port=6
  wires:
  pgas/1 -> Product/1
  Product/1 -> Add/2
  Constant1/1 -> Product1/4
  Constant2/1 -> Product1/5
  Product1/1 -> Gain/1
  Gain/1 -> Add/1
  Constant3/1 -> Product/2
  Add/1 -> X/1
  Product2/1 -> Gain1/1
  Constant6/1 -> Product2/4
  [modV] -> Product2/3
  Constant5/1 -> Product2/5
  Gain1/1 -> Y/1
  [modV] -> Product3/3
  Constant9/1 -> Product3/4
  Constant8/1 -> Product3/5
  Product3/1 -> Gain2/1
  Gain2/1 -> Add1/1
  Product4/1 -> Gain3/1
  Gain3/1 -> Add1/2
  [modV] -> Square/1
  Square/1 -> Product4/2
  Constant12/1 -> Product4/3
  Add1/1 -> Z/1
  Square1/1 -> Product5/2
  [modV] -> Square1/1
  Constant14/1 -> Product5/3
  Constant15/1 -> Product5/4
  Constant16/1 -> Product6/1
  Constant18/1 -> Product7/1
  deltaa/1 -> Product7/2
  Product7/1 -> Add2/2
  Product6/1 -> Add2/1
  Add2/1 -> Product5/5
  Product5/1 -> Gain4/1
  Gain4/1 -> L/1
  Product8/1 -> Gain5/1
  [modV] -> Product8/2
  Constant20/1 -> Product8/3
  Constant21/1 -> Product8/4
  Constant22/1 -> Product9/1
  Constant24/1 -> Product10/1
  [modV] -> Product10/3
  Constant27/1 -> Product11/1
  Product9/1 -> Add3/1
  Product10/1 -> Add3/2
  Product11/1 -> Add3/3
  Add3/1 -> Product8/5
  Gain5/1 -> M/1
  deltae/1 -> Product11/3
  W/1 -> [W]
  [W] -> Product3/2
  [W] -> Product9/2
  P/1 -> Product6/2
  Q/1 -> Product10/2
  Product12/1 -> Gain6/1
  ro/1 -> Product12/1, Product8/1, Product5/1, Product4/1, Product3/1, Product2/1, Product1/2
  Constant23/1 -> Product12/3
  Constant25/1 -> Product12/4
  [V] -> Product15/2
  Constant30/1 -> Product13/1
  Product15/1 -> Add4/1
  Product14/1 -> Add4/3
  Constant32/1 -> Product14/1
  [modV] -> Product13/3
  [modV] -> Product14/2
  Constant29/1 -> Product15/1
  Product13/1 -> Add4/2
  Add4/1 -> Product12/5
  R/1 -> Product13/2
  deltar/1 -> Product14/3
  Gain6/1 -> N/1
  V/1 -> [V]
  [V] -> Product2/2
  U/1 -> [U]
  [U] -> Product1/1
  [W] -> Square4/1
  [V] -> Square3/1
  [U] -> Square2/1
  Square2/1 -> Add5/1
  Square3/1 -> Add5/2
  Square4/1 -> Add5/3
  Add5/1 -> [modV]
  [modV] -> Product1/3
  Constant4/1 -> Power/2
  Constant/1 -> Power/1
  Power/1 -> Add6/2
  [U] -> Add6/1
  Add6/1 -> Divide/2
  [W] -> Divide/1
  Divide/1 -> Trigonometric Function/1
  Trigonometric Function/1 -> [alpha]
  [alpha] -> Product16/1
  Constant7/1 -> Product16/2
  Pi/1 -> Product16/3
  Product16/1 -> [CL]
  [CL] -> Product4/4
  [modV] -> Product12/2
  [modV] -> Product11/2

== system eom/rang ==
  P : Inport
  Q : Inport  Port=2
  R : Inport  Port=3
  phi : Inport  Port=4
  theta : Inport  Port=5
  psi : Inport  Port=6
  Add : Sum
  Add1 : Sum
  Add2 : Sum  Inputs=+-
  Add3 : Sum
  Constant : Constant
  Divide : Product  Inputs=*/
  Product{1..8} (8 alike) : Product
  Trigonometric Function : Trigonometry
  Trigonometric Function{1,3,6..7} (4 alike) : Trigonometry  Operator=cos
  Trigonometric Function2 : Trigonometry  Operator=tan
  Trigonometric Function4 : Trigonometry
  Trigonometric Function5 : Trigonometry
  phidot : Outport
  thetadot : Outport  Port=2
  psidot : Outport  Port=3
  wires:
  P/1 -> [P]
  Q/1 -> [Q]
  R/1 -> [R]
  phi/1 -> [phi]
  theta/1 -> [theta]
  psi/1 -> [psi]
  [P] -> Add/1
  [Q] -> Product1/1
  [phi] -> Trigonometric Function/1
  Trigonometric Function/1 -> Product1/2
  Product1/1 -> Add1/1
  Trigonometric Function1/1 -> Product2/2
  [phi] -> Trigonometric Function1/1
  [R] -> Product2/1
  Product2/1 -> Add1/2
  Add1/1 -> Product3/1
  Product3/1 -> Add/2
  [theta] -> Trigonometric Function2/1
  Trigonometric Function2/1 -> Product3/2
  Add/1 -> phidot/1
  Product5/1 -> Add2/2
  Trigonometric Function3/1 -> Product4/2
  [Q] -> Product4/1
  [R] -> Product5/1
  [phi] -> Trigonometric Function4/1
  Trigonometric Function4/1 -> Product5/2
  [phi] -> Trigonometric Function3/1
  Product4/1 -> Add2/1
  Add2/1 -> thetadot/1
  Trigonometric Function5/1 -> Product6/2
  [theta] -> Trigonometric Function7/1
  [phi] -> Trigonometric Function5/1
  Product7/1 -> Add3/2
  [Q] -> Product6/1
  [phi] -> Trigonometric Function6/1
  Trigonometric Function6/1 -> Product7/2
  Add3/1 -> Product8/1
  [R] -> Product7/1
  Product6/1 -> Add3/1
  Product8/1 -> psidot/1
  Constant/1 -> Divide/1
  Trigonometric Function7/1 -> Divide/2
  Divide/1 -> Product8/2

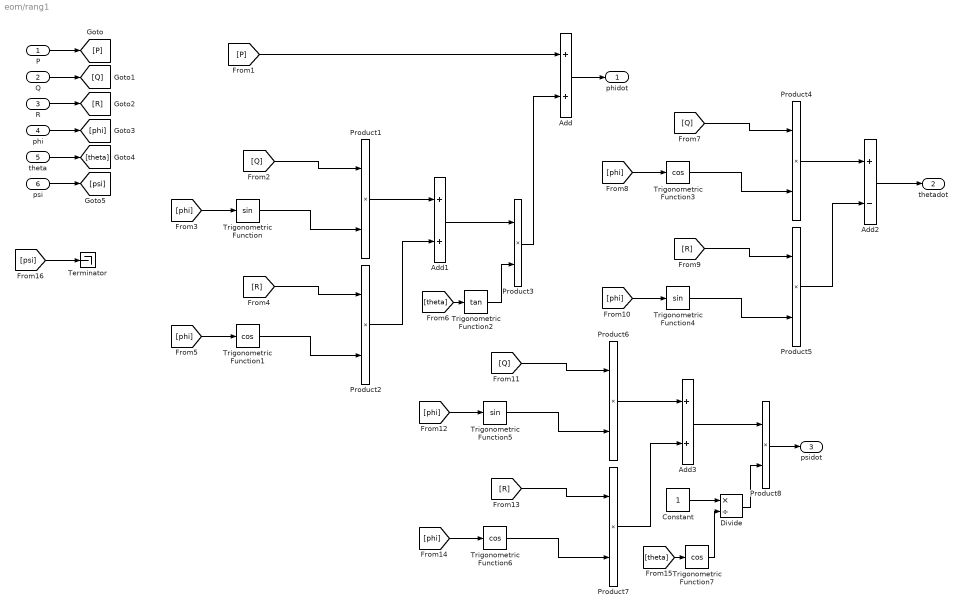
== system eom/rang1 ==
  P : Inport
  Q : Inport  Port=2
  R : Inport  Port=3
  phi : Inport  Port=4
  theta : Inport  Port=5
  psi : Inport  Port=6
  Add : Sum
  Add1 : Sum
  Add2 : Sum  Inputs=+-
  Add3 : Sum
  Constant : Constant
  Divide : Product  Inputs=*/
  Product{1..8} (8 alike) : Product
  Terminator : Terminator
  Trigonometric Function : Trigonometry
  Trigonometric Function{1,3,6..7} (4 alike) : Trigonometry  Operator=cos
  Trigonometric Function2 : Trigonometry  Operator=tan
  Trigonometric Function4 : Trigonometry
  Trigonometric Function5 : Trigonometry
  phidot : Outport
  thetadot : Outport  Port=2
  psidot : Outport  Port=3
  wires:
  P/1 -> [P]
  Q/1 -> [Q]
  R/1 -> [R]
  phi/1 -> [phi]
  theta/1 -> [theta]
  psi/1 -> [psi]
  [P] -> Add/1
  [Q] -> Product1/1
  [phi] -> Trigonometric Function/1
  Trigonometric Function/1 -> Product1/2
  Product1/1 -> Add1/1
  Trigonometric Function1/1 -> Product2/2
  [phi] -> Trigonometric Function1/1
  [R] -> Product2/1
  Product2/1 -> Add1/2
  Add1/1 -> Product3/1
  Product3/1 -> Add/2
  [theta] -> Trigonometric Function2/1
  Trigonometric Function2/1 -> Product3/2
  Add/1 -> phidot/1
  Product5/1 -> Add2/2
  Trigonometric Function3/1 -> Product4/2
  [Q] -> Product4/1
  [R] -> Product5/1
  [phi] -> Trigonometric Function4/1
  Trigonometric Function4/1 -> Product5/2
  [phi] -> Trigonometric Function3/1
  Product4/1 -> Add2/1
  Add2/1 -> thetadot/1
  Trigonometric Function5/1 -> Product6/2
  [theta] -> Trigonometric Function7/1
  [phi] -> Trigonometric Function5/1
  Product7/1 -> Add3/2
  [Q] -> Product6/1
  [phi] -> Trigonometric Function6/1
  Trigonometric Function6/1 -> Product7/2
  Add3/1 -> Product8/1
  [R] -> Product7/1
  Product6/1 -> Add3/1
  Product8/1 -> psidot/1
  Constant/1 -> Divide/1
  Trigonometric Function7/1 -> Divide/2
  Divide/1 -> Product8/2
  [psi] -> Terminator/1

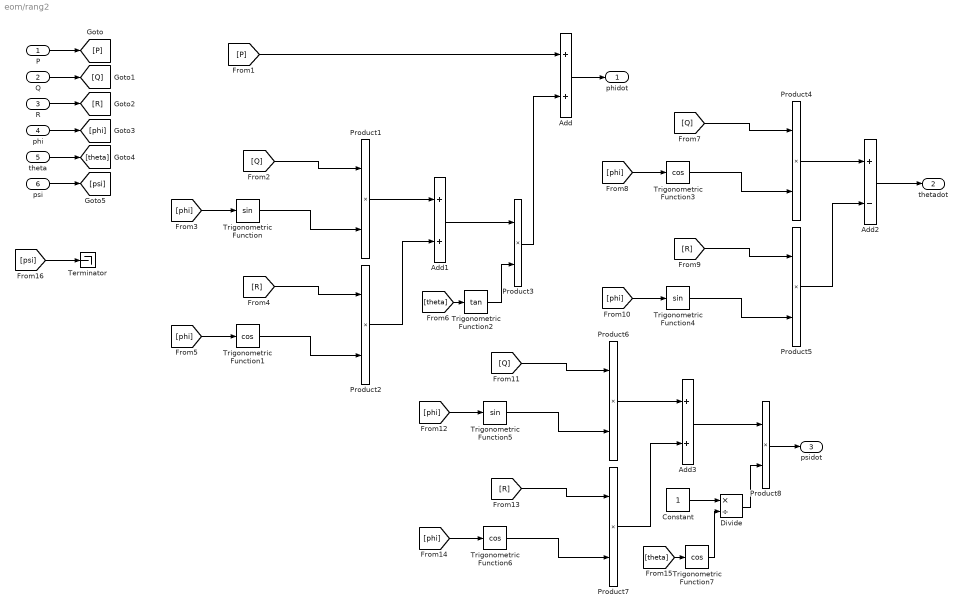
== system eom/rang2 ==
  P : Inport
  Q : Inport  Port=2
  R : Inport  Port=3
  phi : Inport  Port=4
  theta : Inport  Port=5
  psi : Inport  Port=6
  Add : Sum
  Add1 : Sum
  Add2 : Sum  Inputs=+-
  Add3 : Sum
  Constant : Constant
  Divide : Product  Inputs=*/
  Product{1..8} (8 alike) : Product
  Terminator : Terminator
  Trigonometric Function : Trigonometry
  Trigonometric Function{1,3,6..7} (4 alike) : Trigonometry  Operator=cos
  Trigonometric Function2 : Trigonometry  Operator=tan
  Trigonometric Function4 : Trigonometry
  Trigonometric Function5 : Trigonometry
  phidot : Outport
  thetadot : Outport  Port=2
  psidot : Outport  Port=3
  wires:
  P/1 -> [P]
  Q/1 -> [Q]
  R/1 -> [R]
  phi/1 -> [phi]
  theta/1 -> [theta]
  psi/1 -> [psi]
  [P] -> Add/1
  [Q] -> Product1/1
  [phi] -> Trigonometric Function/1
  Trigonometric Function/1 -> Product1/2
  Product1/1 -> Add1/1
  Trigonometric Function1/1 -> Product2/2
  [phi] -> Trigonometric Function1/1
  [R] -> Product2/1
  Product2/1 -> Add1/2
  Add1/1 -> Product3/1
  Product3/1 -> Add/2
  [theta] -> Trigonometric Function2/1
  Trigonometric Function2/1 -> Product3/2
  Add/1 -> phidot/1
  Product5/1 -> Add2/2
  Trigonometric Function3/1 -> Product4/2
  [Q] -> Product4/1
  [R] -> Product5/1
  [phi] -> Trigonometric Function4/1
  Trigonometric Function4/1 -> Product5/2
  [phi] -> Trigonometric Function3/1
  Product4/1 -> Add2/1
  Add2/1 -> thetadot/1
  Trigonometric Function5/1 -> Product6/2
  [theta] -> Trigonometric Function7/1
  [phi] -> Trigonometric Function5/1
  Product7/1 -> Add3/2
  [Q] -> Product6/1
  [phi] -> Trigonometric Function6/1
  Trigonometric Function6/1 -> Product7/2
  Add3/1 -> Product8/1
  [R] -> Product7/1
  Product6/1 -> Add3/1
  Product8/1 -> psidot/1
  Constant/1 -> Divide/1
  Trigonometric Function7/1 -> Divide/2
  Divide/1 -> Product8/2
  [psi] -> Terminator/1

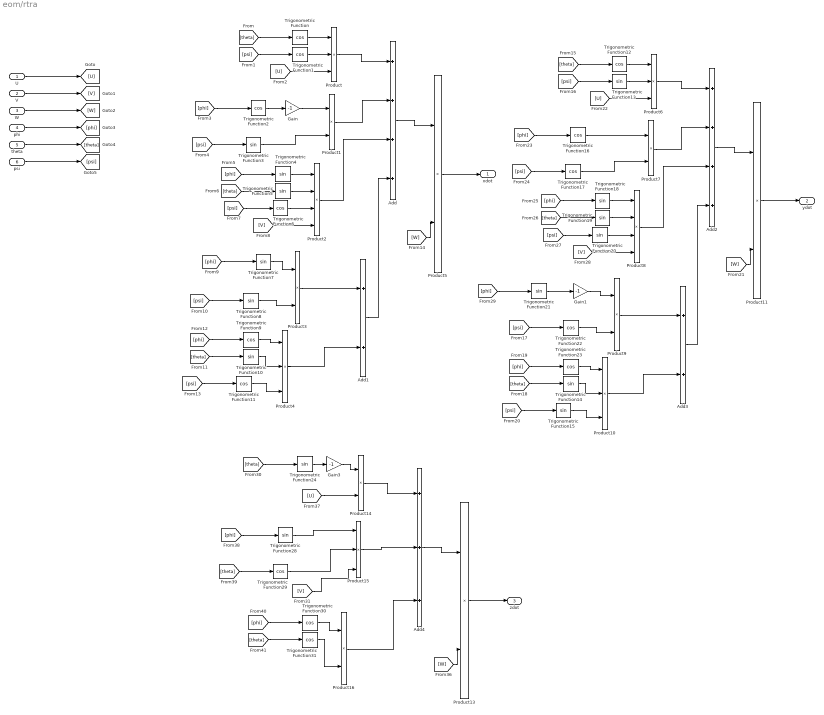
== system eom/rtra ==
  U : Inport
  V : Inport  Port=2
  W : Inport  Port=3
  phi : Inport  Port=4
  theta : Inport  Port=5
  psi : Inport  Port=6
  Add : Sum  Inputs=++++
  Add1 : Sum
  Add2 : Sum  Inputs=++++
  Add3 : Sum
  Add4 : Sum  Inputs=+++
  Gain : Gain  Gain=-1
  Gain1 : Gain  Gain=-1
  Gain3 : Gain  Gain=-1
  Product{,4,6,10,15} (5 alike) : Product  Inputs=3
  Product{1,3,5,7,9,11,13..14,16} (9 alike) : Product
  Product2 : Product  Inputs=4
  Product8 : Product  Inputs=4
  Trigonometric Function{,1..2,6,9,11..12,16..17,22..23,29..31} (14 alike) : Trigonometry  Operator=cos
  Trigonometric Function{3..5,7..8,10,13..15,18..21,24,28} (15 alike) : Trigonometry
  xdot : Outport
  ydot : Outport  Port=2
  zdot : Outport  Port=3
  wires:
  U/1 -> [U]
  V/1 -> [V]
  W/1 -> [W]
  phi/1 -> [phi]
  theta/1 -> [theta]
  psi/1 -> [psi]
  [theta] -> Trigonometric Function/1
  Trigonometric Function/1 -> Product/1
  [psi] -> Trigonometric Function1/1
  Trigonometric Function1/1 -> Product/2
  [U] -> Product/3
  Product/1 -> Add/1
  [phi] -> Trigonometric Function2/1
  Trigonometric Function2/1 -> Gain/1
  [psi] -> Trigonometric Function3/1
  Gain/1 -> Product1/1
  Trigonometric Function3/1 -> Product1/2
  [theta] -> Trigonometric Function5/1
  Trigonometric Function5/1 -> Product2/2
  [phi] -> Trigonometric Function4/1
  Trigonometric Function4/1 -> Product2/1
  [V] -> Product2/4
  Product2/1 -> Add/3
  [psi] -> Trigonometric Function6/1
  Trigonometric Function6/1 -> Product2/3
  [psi] -> Trigonometric Function8/1
  Trigonometric Function7/1 -> Product3/1
  Trigonometric Function8/1 -> Product3/2
  [phi] -> Trigonometric Function7/1
  Trigonometric Function10/1 -> Product4/2
  Trigonometric Function9/1 -> Product4/1
  [theta] -> Trigonometric Function10/1
  [phi] -> Trigonometric Function9/1
  Add1/1 -> Add/4
  Product3/1 -> Add1/1
  Product4/1 -> Add1/2
  Trigonometric Function11/1 -> Product4/3
  [psi] -> Trigonometric Function11/1
  [W] -> Product5/2
  Add/1 -> Product5/1
  Product5/1 -> xdot/1
  [psi] -> Trigonometric Function13/1
  Trigonometric Function16/1 -> Product7/1
  [V] -> Product8/4
  Trigonometric Function13/1 -> Product6/2
  [psi] -> Trigonometric Function20/1
  [psi] -> Trigonometric Function17/1
  Add2/1 -> Product11/1
  Trigonometric Function20/1 -> Product8/3
  Trigonometric Function18/1 -> Product8/1
  [theta] -> Trigonometric Function19/1
  Product8/1 -> Add2/3
  Trigonometric Function17/1 -> Product7/2
  Trigonometric Function21/1 -> Gain1/1
  Product10/1 -> Add3/2
  [phi] -> Trigonometric Function23/1
  [theta] -> Trigonometric Function12/1
  [theta] -> Trigonometric Function14/1
  Trigonometric Function23/1 -> Product10/1
  Trigonometric Function14/1 -> Product10/2
  Product6/1 -> Add2/1
  Product11/1 -> ydot/1
  [psi] -> Trigonometric Function15/1
  Product9/1 -> Add3/1
  Trigonometric Function15/1 -> Product10/3
  [W] -> Product11/2
  Trigonometric Function22/1 -> Product9/2
  [phi] -> Trigonometric Function16/1
  [phi] -> Trigonometric Function21/1
  Product7/1 -> Add2/2
  Add3/1 -> Add2/4
  Trigonometric Function12/1 -> Product6/1
  Trigonometric Function19/1 -> Product8/2
  [phi] -> Trigonometric Function18/1
  [U] -> Product6/3
  [psi] -> Trigonometric Function22/1
  Gain1/1 -> Product9/1
  Trigonometric Function31/1 -> Product16/2
  [phi] -> Trigonometric Function28/1
  [W] -> Product13/2
  Product14/1 -> Add4/1
  Trigonometric Function28/1 -> Product15/1
  [theta] -> Trigonometric Function24/1
  Product13/1 -> zdot/1
  Product15/1 -> Add4/2
  Trigonometric Function29/1 -> Product15/2
  Product16/1 -> Add4/3
  Trigonometric Function30/1 -> Product16/1
  [theta] -> Trigonometric Function31/1
  Add4/1 -> Product13/1
  [theta] -> Trigonometric Function29/1
  [phi] -> Trigonometric Function30/1
  Trigonometric Function24/1 -> Gain3/1
  Gain3/1 -> Product14/1
  [U] -> Product14/2
  [V] -> Product15/3
  Product1/1 -> Add/2
